simulink model "PMSM_CascadedMPC"  (R2025b)
settings: Solver=ode3  StartTime=0.0  StopTime=12  FixedStep=5e-6  MaxStep=1e-4  RelTol=1e-3
PreLoadFcn:
  | run('params_pmsm_inverter')
undefined symbols (not defined in the file): B_fric, J, Ld, Lq, pp, PsiPM, Rs, Ts_ctrl, Ts_sim, Vdc
libraries: nesl_utility x16, fl_lib x11, ee_lib x8, simulink x1, sdl_lib x1
(part 2 of 2)

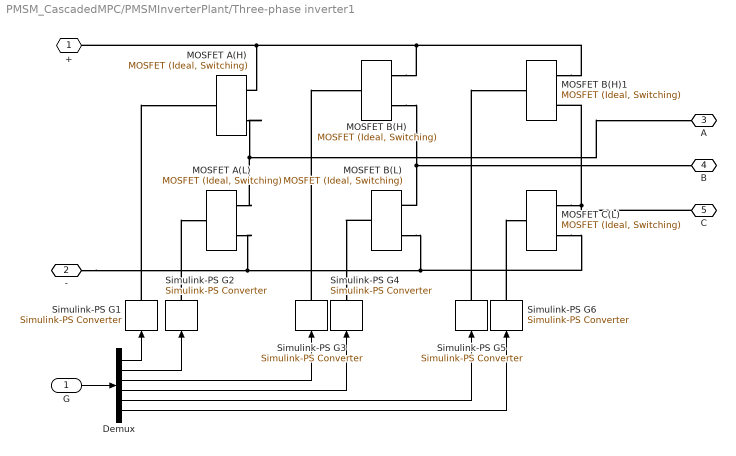
== system PMSM_CascadedMPC/PMSMInverterPlant/Three-phase inverter1 ==
  G : Inport
  Demux : Demux  Outputs=6
  MOSFET A(H) : ee_lib/Semiconductors & Converters/MOSFET (Ideal, Switching)  port_option=ee.enum.controlport.ps  Rds=0.01 Ohm  Goff=1e-6 1/Ohm  Vth=0.5 V  diode_param=ee.enum.semiconductors.protectionDiode.nodynamics  diode_Vf=0.8 V  diode_Ron=0.001 Ohm  diode_Goff=1e-5 1/Ohm  diode_C=50e-9 F  diode_iRM=-235 A  diode_iF=300 A  diode_idot=-50 A/us  diode_trr_param=ee.enum.converters.diodeReverseParam.trr_factor  diode_trr_factor=3  diode_trr=15 us  diode_Qrr=1500 s*uA  ids_specify=off  ids_priority=None  ids=0 A  ids_nominal_specify=off  ids_nominal_value=1  ids_nominal_unit=A  vds_specify=off  vds_priority=None  vds=0 V  vds_nominal_specify=off  vds_nominal_value=1  vds_nominal_unit=V  vgs_specify=off  vgs_priority=None  vgs=0 V  vgs_nominal_specify=off  vgs_nominal_value=1  vgs_nominal_unit=V  thermal_loss_option=ee.enum.converters.thermalLossOption.constantvalues  Von_data=[0, 1.8, 3.2, 6, 10, 16; 0, 2, 5.5, 9.5, 15, 25] V  Tj=[298.15, 448.15] K  Iout_data=[0, 20, 40, 60, 80, 100] A  Eon_data=[0, 55.04, 124.57, 235.53, 362.12; 0, 71.25, 161.25, 304.88, 468.75] * 1e-6 J  Eoff_data=[0, 18, 30, 56.1, 76.5; 0, 22.5, 37.5, 70.13, 95.63] * 1e-6 J  Eon_data_3D=[zeros(2, 5, 3)] J  Eoff_data_3D=[zeros(2, 5, 3)] J  Tj_loss=[298.15, 448.15] K  Iout_data_loss=[0, 10, 20, 30, 40] A  tabulateWithVds=false  Vds_loss=[0, 150, 300] V  Eon_scalar=22.86e-3 J  Eoff_scalar=17.14e-3 J  Voff=800 V  Iout_scalar=600 A  useCurrentFromPreviousCycle=false  useVoltageFromPreviousCycle=false  diodeModelType=ee.enum.converters.diodeModelType.pwl  diodeTableType=ee.enum.diode.tableType.IfMat  diode_ReverseIVType=ee.enum.diode.diodeReverseIV.constant  diode_IfMat=[.07, .12, .19, 1.75, 4.24, 7.32, 11.2; .16, .3, .72, 2.14, 4.02, 6.35, 9.12] A  diode_VfMat=[.9, 1.15, 1.25, 1.5, 1.75, 2.17, 2.6, 2.85; .58, .68, .75, 1.1, 1.38, 1.77, 2.27, 2.7] V  diode_TjVec=[25, 125] degC  diode_VfVec=[.5, .7, .9, 1.3, 1.7, 2.1, 2.5] V  diode_IfVec=[.1, .2, .5, 1, 2, 4, 7, 10] A  diode_IrMat=[1e-06, 2e-06, 5e-06, 1e-05, 2.5e-05, 5e-05, .0001; 2e-06, 5e-06, 1e-05, 4e-05, 8e-05, .0002, .0005] A  diode_VrMat=[10, 100, 200, 250, 300, 325, 350; 10, 70, 160, 220, 270, 300, 320] V  diode_VrVec=[10, 20, 40, 50, 70, 80, 100] V  diode_IrVec=[1e-06, 2e-06, 5e-06, 1e-05, 2e-05, 5e-05, .0001] A  diode_Vr=-600 V  diode_Ls=150 nH  diode_Erec=0.03 J  diode_rec_loss_model=ee.enum.diode.reverseRecoveryModel.fixed  diode_ErecVal=0 J  diode_scaleWithIandV=true  diode_ErecMat=zeros(2, 3) J  diode_TjrecVec=[298.15, 398.15] K  diode_IfrecVec=[.1, 1, 10] A  diode_IrecVal=10 A  diode_VrecVal=10 V  diode_tFilter=1 / 1000 / 100 s  separateThermalPortForDiode=false  thermal_network_parameterization=ee.enum.thermalNetworkTopology.junctionCase  Rth=[.03, .2] K/W  Rth_Cauer=[.03, .1, .2] K/W  Rth_Foster=[.08, .14, .22, .16] K/W  thermal_mass_parameterization=ee.enum.thermalNetwork.thermalmass  thermal_mass=[3, 25] J/K  thermal_mass_Cauer=[3, 10, 25] J/K  thermal_mass_Foster=[.001, .005, .05, .5] J/K  thermal_time_constant=[.1, 5] s  thermal_time_constant_Cauer=[.1, 1, 5] s  thermal_time_constant_Foster=[7e-05, .0007, .01, .08] s  thermal_mass_initial_temperatures=[25, 25] degC  thermal_mass_initial_temperatures_Cauer=[25, 25, 25] degC  junction_thermal_mass=5 J/K  Tvec_initial_Foster=[25, 25, 25, 25] degC  RthDiode=[.03, .2] K/W  RthCauerDiode=[.03, .1, .2] K/W  RthFosterDiode=[.03, .2] K/W  thermalMassDiode=[3, 25] J/K  thermalMassCauerDiode=[3, 10, 25] J/K  thermalMassFosterDiode=[33, 50] J/K  thermalTauDiode=[.1, 5] s  thermalTauCauerDiode=[.1, 1, 5] s  thermalTauFosterDiode=[1, 10] s  thermalMassInitTempDiode=[25, 25] degC  thermalMassInitTempCauerDiode=[25, 25, 25] degC  junctionthermalMassDiode=0.1 J/K  TVecInitialFosterDiode=[25, 25, 25, 25] degC  no_thermal_network=0  mosfet_junction_temperature_specify=on  mosfet_junction_temperature_priority=None  mosfet_junction_temperature=25 degC  mosfet_junction_temperature_nominal_specify=off  mosfet_junction_temperature_nominal_value=1  mosfet_junction_temperature_nominal_unit=degC  diode_junction_temperature_specify=off  diode_junction_temperature_priority=None  diode_junction_temperature=25 degC  diode_junction_temperature_nominal_specify=off  diode_junction_temperature_nominal_value=1  diode_junction_temperature_nominal_unit=degC  Qj_specify=off  Qj_priority=None  Qj=0 W  Qj_nominal_specify=off  Qj_nominal_value=1  Qj_nominal_unit=W  accumulatedSwitchingLosses_specify=off  accumulatedSwitchingLosses_priority=None  accumulatedSwitchingLosses=0 J
  MOSFET A(L) : ee_lib/Semiconductors & Converters/MOSFET (Ideal, Switching)  port_option=ee.enum.controlport.ps  Rds=0.01 Ohm  Goff=1e-6 1/Ohm  Vth=0.5 V  diode_param=ee.enum.semiconductors.protectionDiode.nodynamics  diode_Vf=0.8 V  diode_Ron=0.001 Ohm  diode_Goff=1e-5 1/Ohm  diode_C=50e-9 F  diode_iRM=-235 A  diode_iF=300 A  diode_idot=-50 A/us  diode_trr_param=ee.enum.converters.diodeReverseParam.trr_factor  diode_trr_factor=3  diode_trr=15 us  diode_Qrr=1500 s*uA  ids_specify=off  ids_priority=None  ids=0 A  ids_nominal_specify=off  ids_nominal_value=1  ids_nominal_unit=A  vds_specify=off  vds_priority=None  vds=0 V  vds_nominal_specify=off  vds_nominal_value=1  vds_nominal_unit=V  vgs_specify=off  vgs_priority=None  vgs=0 V  vgs_nominal_specify=off  vgs_nominal_value=1  vgs_nominal_unit=V  thermal_loss_option=ee.enum.converters.thermalLossOption.constantvalues  Von_data=[0, 1.8, 3.2, 6, 10, 16; 0, 2, 5.5, 9.5, 15, 25] V  Tj=[298.15, 448.15] K  Iout_data=[0, 20, 40, 60, 80, 100] A  Eon_data=[0, 55.04, 124.57, 235.53, 362.12; 0, 71.25, 161.25, 304.88, 468.75] * 1e-6 J  Eoff_data=[0, 18, 30, 56.1, 76.5; 0, 22.5, 37.5, 70.13, 95.63] * 1e-6 J  Eon_data_3D=[zeros(2, 5, 3)] J  Eoff_data_3D=[zeros(2, 5, 3)] J  Tj_loss=[298.15, 448.15] K  Iout_data_loss=[0, 10, 20, 30, 40] A  tabulateWithVds=false  Vds_loss=[0, 150, 300] V  Eon_scalar=22.86e-3 J  Eoff_scalar=17.14e-3 J  Voff=300 V  Iout_scalar=600 A  useCurrentFromPreviousCycle=false  useVoltageFromPreviousCycle=false  diodeModelType=ee.enum.converters.diodeModelType.pwl  diodeTableType=ee.enum.diode.tableType.IfMat  diode_ReverseIVType=ee.enum.diode.diodeReverseIV.constant  diode_IfMat=[.07, .12, .19, 1.75, 4.24, 7.32, 11.2; .16, .3, .72, 2.14, 4.02, 6.35, 9.12] A  diode_VfMat=[.9, 1.15, 1.25, 1.5, 1.75, 2.17, 2.6, 2.85; .58, .68, .75, 1.1, 1.38, 1.77, 2.27, 2.7] V  diode_TjVec=[25, 125] degC  diode_VfVec=[.5, .7, .9, 1.3, 1.7, 2.1, 2.5] V  diode_IfVec=[.1, .2, .5, 1, 2, 4, 7, 10] A  diode_IrMat=[1e-06, 2e-06, 5e-06, 1e-05, 2.5e-05, 5e-05, .0001; 2e-06, 5e-06, 1e-05, 4e-05, 8e-05, .0002, .0005] A  diode_VrMat=[10, 100, 200, 250, 300, 325, 350; 10, 70, 160, 220, 270, 300, 320] V  diode_VrVec=[10, 20, 40, 50, 70, 80, 100] V  diode_IrVec=[1e-06, 2e-06, 5e-06, 1e-05, 2e-05, 5e-05, .0001] A  diode_Vr=-600 V  diode_Ls=150 nH  diode_Erec=0.03 J  diode_rec_loss_model=ee.enum.diode.reverseRecoveryModel.fixed  diode_ErecVal=0 J  diode_scaleWithIandV=true  diode_ErecMat=zeros(2, 3) J  diode_TjrecVec=[298.15, 398.15] K  diode_IfrecVec=[.1, 1, 10] A  diode_IrecVal=10 A  diode_VrecVal=10 V  diode_tFilter=1 / 1000 / 100 s  separateThermalPortForDiode=false  thermal_network_parameterization=ee.enum.thermalNetworkTopology.external  Rth=[.03, .2] K/W  Rth_Cauer=[.03, .1, .2] K/W  Rth_Foster=[.08, .14, .22, .16] K/W  thermal_mass_parameterization=ee.enum.thermalNetwork.timeconstant  thermal_mass=[3, 25] J/K  thermal_mass_Cauer=[3, 10, 25] J/K  thermal_mass_Foster=[.001, .005, .05, .5] J/K  thermal_time_constant=[.1, 5] s  thermal_time_constant_Cauer=[.1, 1, 5] s  thermal_time_constant_Foster=[7e-05, .0007, .01, .08] s  thermal_mass_initial_temperatures=[25, 25] degC  thermal_mass_initial_temperatures_Cauer=[25, 25, 25] degC  junction_thermal_mass=0.1 J/K  Tvec_initial_Foster=[25, 25, 25, 25] degC  RthDiode=[.03, .2] K/W  RthCauerDiode=[.03, .1, .2] K/W  RthFosterDiode=[.03, .2] K/W  thermalMassDiode=[3, 25] J/K  thermalMassCauerDiode=[3, 10, 25] J/K  thermalMassFosterDiode=[33, 50] J/K  thermalTauDiode=[.1, 5] s  thermalTauCauerDiode=[.1, 1, 5] s  thermalTauFosterDiode=[1, 10] s  thermalMassInitTempDiode=[25, 25] degC  thermalMassInitTempCauerDiode=[25, 25, 25] degC  junctionthermalMassDiode=0.1 J/K  TVecInitialFosterDiode=[25, 25, 25, 25] degC  no_thermal_network=0  mosfet_junction_temperature_specify=off  mosfet_junction_temperature_priority=None  mosfet_junction_temperature=25 degC  mosfet_junction_temperature_nominal_specify=off  mosfet_junction_temperature_nominal_value=1  mosfet_junction_temperature_nominal_unit=degC  diode_junction_temperature_specify=off  diode_junction_temperature_priority=None  diode_junction_temperature=25 degC  diode_junction_temperature_nominal_specify=off  diode_junction_temperature_nominal_value=1  diode_junction_temperature_nominal_unit=degC  Qj_specify=off  Qj_priority=None  Qj=0 W  Qj_nominal_specify=off  Qj_nominal_value=1  Qj_nominal_unit=W  accumulatedSwitchingLosses_specify=off  accumulatedSwitchingLosses_priority=None  accumulatedSwitchingLosses=0 J
  MOSFET B(H) : ee_lib/Semiconductors & Converters/MOSFET (Ideal, Switching)  port_option=ee.enum.controlport.ps  Rds=0.01 Ohm  Goff=1e-6 1/Ohm  Vth=0.5 V  diode_param=ee.enum.semiconductors.protectionDiode.nodynamics  diode_Vf=0.8 V  diode_Ron=0.001 Ohm  diode_Goff=1e-5 1/Ohm  diode_C=50e-9 F  diode_iRM=-235 A  diode_iF=300 A  diode_idot=-50 A/us  diode_trr_param=ee.enum.converters.diodeReverseParam.trr_factor  diode_trr_factor=3  diode_trr=15 us  diode_Qrr=1500 s*uA  ids_specify=off  ids_priority=None  ids=0 A  ids_nominal_specify=off  ids_nominal_value=1  ids_nominal_unit=A  vds_specify=off  vds_priority=None  vds=0 V  vds_nominal_specify=off  vds_nominal_value=1  vds_nominal_unit=V  vgs_specify=off  vgs_priority=None  vgs=0 V  vgs_nominal_specify=off  vgs_nominal_value=1  vgs_nominal_unit=V  thermal_loss_option=ee.enum.converters.thermalLossOption.constantvalues  Von_data=[0, 1.8, 3.2, 6, 10, 16; 0, 2, 5.5, 9.5, 15, 25] V  Tj=[298.15, 448.15] K  Iout_data=[0, 20, 40, 60, 80, 100] A  Eon_data=[0, 55.04, 124.57, 235.53, 362.12; 0, 71.25, 161.25, 304.88, 468.75] * 1e-6 J  Eoff_data=[0, 18, 30, 56.1, 76.5; 0, 22.5, 37.5, 70.13, 95.63] * 1e-6 J  Eon_data_3D=[zeros(2, 5, 3)] J  Eoff_data_3D=[zeros(2, 5, 3)] J  Tj_loss=[298.15, 448.15] K  Iout_data_loss=[0, 10, 20, 30, 40] A  tabulateWithVds=false  Vds_loss=[0, 150, 300] V  Eon_scalar=22.86e-3 J  Eoff_scalar=17.14e-3 J  Voff=300 V  Iout_scalar=600 A  useCurrentFromPreviousCycle=false  useVoltageFromPreviousCycle=false  diodeModelType=ee.enum.converters.diodeModelType.pwl  diodeTableType=ee.enum.diode.tableType.IfMat  diode_ReverseIVType=ee.enum.diode.diodeReverseIV.constant  diode_IfMat=[.07, .12, .19, 1.75, 4.24, 7.32, 11.2; .16, .3, .72, 2.14, 4.02, 6.35, 9.12] A  diode_VfMat=[.9, 1.15, 1.25, 1.5, 1.75, 2.17, 2.6, 2.85; .58, .68, .75, 1.1, 1.38, 1.77, 2.27, 2.7] V  diode_TjVec=[25, 125] degC  diode_VfVec=[.5, .7, .9, 1.3, 1.7, 2.1, 2.5] V  diode_IfVec=[.1, .2, .5, 1, 2, 4, 7, 10] A  diode_IrMat=[1e-06, 2e-06, 5e-06, 1e-05, 2.5e-05, 5e-05, .0001; 2e-06, 5e-06, 1e-05, 4e-05, 8e-05, .0002, .0005] A  diode_VrMat=[10, 100, 200, 250, 300, 325, 350; 10, 70, 160, 220, 270, 300, 320] V  diode_VrVec=[10, 20, 40, 50, 70, 80, 100] V  diode_IrVec=[1e-06, 2e-06, 5e-06, 1e-05, 2e-05, 5e-05, .0001] A  diode_Vr=-600 V  diode_Ls=150 nH  diode_Erec=0.03 J  diode_rec_loss_model=ee.enum.diode.reverseRecoveryModel.fixed  diode_ErecVal=0 J  diode_scaleWithIandV=true  diode_ErecMat=zeros(2, 3) J  diode_TjrecVec=[298.15, 398.15] K  diode_IfrecVec=[.1, 1, 10] A  diode_IrecVal=10 A  diode_VrecVal=10 V  diode_tFilter=1 / 1000 / 100 s  separateThermalPortForDiode=false  thermal_network_parameterization=ee.enum.thermalNetworkTopology.external  Rth=[.03, .2] K/W  Rth_Cauer=[.03, .1, .2] K/W  Rth_Foster=[.08, .14, .22, .16] K/W  thermal_mass_parameterization=ee.enum.thermalNetwork.timeconstant  thermal_mass=[3, 25] J/K  thermal_mass_Cauer=[3, 10, 25] J/K  thermal_mass_Foster=[.001, .005, .05, .5] J/K  thermal_time_constant=[.1, 5] s  thermal_time_constant_Cauer=[.1, 1, 5] s  thermal_time_constant_Foster=[7e-05, .0007, .01, .08] s  thermal_mass_initial_temperatures=[25, 25] degC  thermal_mass_initial_temperatures_Cauer=[25, 25, 25] degC  junction_thermal_mass=0.1 J/K  Tvec_initial_Foster=[25, 25, 25, 25] degC  RthDiode=[.03, .2] K/W  RthCauerDiode=[.03, .1, .2] K/W  RthFosterDiode=[.03, .2] K/W  thermalMassDiode=[3, 25] J/K  thermalMassCauerDiode=[3, 10, 25] J/K  thermalMassFosterDiode=[33, 50] J/K  thermalTauDiode=[.1, 5] s  thermalTauCauerDiode=[.1, 1, 5] s  thermalTauFosterDiode=[1, 10] s  thermalMassInitTempDiode=[25, 25] degC  thermalMassInitTempCauerDiode=[25, 25, 25] degC  junctionthermalMassDiode=0.1 J/K  TVecInitialFosterDiode=[25, 25, 25, 25] degC  no_thermal_network=0  mosfet_junction_temperature_specify=off  mosfet_junction_temperature_priority=None  mosfet_junction_temperature=25 degC  mosfet_junction_temperature_nominal_specify=off  mosfet_junction_temperature_nominal_value=1  mosfet_junction_temperature_nominal_unit=degC  diode_junction_temperature_specify=off  diode_junction_temperature_priority=None  diode_junction_temperature=25 degC  diode_junction_temperature_nominal_specify=off  diode_junction_temperature_nominal_value=1  diode_junction_temperature_nominal_unit=degC  Qj_specify=off  Qj_priority=None  Qj=0 W  Qj_nominal_specify=off  Qj_nominal_value=1  Qj_nominal_unit=W  accumulatedSwitchingLosses_specify=off  accumulatedSwitchingLosses_priority=None  accumulatedSwitchingLosses=0 J
  MOSFET B(H)1 : ee_lib/Semiconductors & Converters/MOSFET (Ideal, Switching)  port_option=ee.enum.controlport.ps  Rds=0.01 Ohm  Goff=1e-6 1/Ohm  Vth=0.5 V  diode_param=ee.enum.semiconductors.protectionDiode.nodynamics  diode_Vf=0.8 V  diode_Ron=0.001 Ohm  diode_Goff=1e-5 1/Ohm  diode_C=50e-9 F  diode_iRM=-235 A  diode_iF=300 A  diode_idot=-50 A/us  diode_trr_param=ee.enum.converters.diodeReverseParam.trr_factor  diode_trr_factor=3  diode_trr=15 us  diode_Qrr=1500 s*uA  ids_specify=off  ids_priority=None  ids=0 A  ids_nominal_specify=off  ids_nominal_value=1  ids_nominal_unit=A  vds_specify=off  vds_priority=None  vds=0 V  vds_nominal_specify=off  vds_nominal_value=1  vds_nominal_unit=V  vgs_specify=off  vgs_priority=None  vgs=0 V  vgs_nominal_specify=off  vgs_nominal_value=1  vgs_nominal_unit=V  thermal_loss_option=ee.enum.converters.thermalLossOption.constantvalues  Von_data=[0, 1.8, 3.2, 6, 10, 16; 0, 2, 5.5, 9.5, 15, 25] V  Tj=[298.15, 448.15] K  Iout_data=[0, 20, 40, 60, 80, 100] A  Eon_data=[0, 55.04, 124.57, 235.53, 362.12; 0, 71.25, 161.25, 304.88, 468.75] * 1e-6 J  Eoff_data=[0, 18, 30, 56.1, 76.5; 0, 22.5, 37.5, 70.13, 95.63] * 1e-6 J  Eon_data_3D=[zeros(2, 5, 3)] J  Eoff_data_3D=[zeros(2, 5, 3)] J  Tj_loss=[298.15, 448.15] K  Iout_data_loss=[0, 10, 20, 30, 40] A  tabulateWithVds=false  Vds_loss=[0, 150, 300] V  Eon_scalar=22.86e-3 J  Eoff_scalar=17.14e-3 J  Voff=300 V  Iout_scalar=600 A  useCurrentFromPreviousCycle=false  useVoltageFromPreviousCycle=false  diodeModelType=ee.enum.converters.diodeModelType.pwl  diodeTableType=ee.enum.diode.tableType.IfMat  diode_ReverseIVType=ee.enum.diode.diodeReverseIV.constant  diode_IfMat=[.07, .12, .19, 1.75, 4.24, 7.32, 11.2; .16, .3, .72, 2.14, 4.02, 6.35, 9.12] A  diode_VfMat=[.9, 1.15, 1.25, 1.5, 1.75, 2.17, 2.6, 2.85; .58, .68, .75, 1.1, 1.38, 1.77, 2.27, 2.7] V  diode_TjVec=[25, 125] degC  diode_VfVec=[.5, .7, .9, 1.3, 1.7, 2.1, 2.5] V  diode_IfVec=[.1, .2, .5, 1, 2, 4, 7, 10] A  diode_IrMat=[1e-06, 2e-06, 5e-06, 1e-05, 2.5e-05, 5e-05, .0001; 2e-06, 5e-06, 1e-05, 4e-05, 8e-05, .0002, .0005] A  diode_VrMat=[10, 100, 200, 250, 300, 325, 350; 10, 70, 160, 220, 270, 300, 320] V  diode_VrVec=[10, 20, 40, 50, 70, 80, 100] V  diode_IrVec=[1e-06, 2e-06, 5e-06, 1e-05, 2e-05, 5e-05, .0001] A  diode_Vr=-600 V  diode_Ls=150 nH  diode_Erec=0.03 J  diode_rec_loss_model=ee.enum.diode.reverseRecoveryModel.fixed  diode_ErecVal=0 J  diode_scaleWithIandV=true  diode_ErecMat=zeros(2, 3) J  diode_TjrecVec=[298.15, 398.15] K  diode_IfrecVec=[.1, 1, 10] A  diode_IrecVal=10 A  diode_VrecVal=10 V  diode_tFilter=1 / 1000 / 100 s  separateThermalPortForDiode=false  thermal_network_parameterization=ee.enum.thermalNetworkTopology.external  Rth=[.03, .2] K/W  Rth_Cauer=[.03, .1, .2] K/W  Rth_Foster=[.08, .14, .22, .16] K/W  thermal_mass_parameterization=ee.enum.thermalNetwork.timeconstant  thermal_mass=[3, 25] J/K  thermal_mass_Cauer=[3, 10, 25] J/K  thermal_mass_Foster=[.001, .005, .05, .5] J/K  thermal_time_constant=[.1, 5] s  thermal_time_constant_Cauer=[.1, 1, 5] s  thermal_time_constant_Foster=[7e-05, .0007, .01, .08] s  thermal_mass_initial_temperatures=[25, 25] degC  thermal_mass_initial_temperatures_Cauer=[25, 25, 25] degC  junction_thermal_mass=0.1 J/K  Tvec_initial_Foster=[25, 25, 25, 25] degC  RthDiode=[.03, .2] K/W  RthCauerDiode=[.03, .1, .2] K/W  RthFosterDiode=[.03, .2] K/W  thermalMassDiode=[3, 25] J/K  thermalMassCauerDiode=[3, 10, 25] J/K  thermalMassFosterDiode=[33, 50] J/K  thermalTauDiode=[.1, 5] s  thermalTauCauerDiode=[.1, 1, 5] s  thermalTauFosterDiode=[1, 10] s  thermalMassInitTempDiode=[25, 25] degC  thermalMassInitTempCauerDiode=[25, 25, 25] degC  junctionthermalMassDiode=0.1 J/K  TVecInitialFosterDiode=[25, 25, 25, 25] degC  no_thermal_network=0  mosfet_junction_temperature_specify=off  mosfet_junction_temperature_priority=None  mosfet_junction_temperature=25 degC  mosfet_junction_temperature_nominal_specify=off  mosfet_junction_temperature_nominal_value=1  mosfet_junction_temperature_nominal_unit=degC  diode_junction_temperature_specify=off  diode_junction_temperature_priority=None  diode_junction_temperature=25 degC  diode_junction_temperature_nominal_specify=off  diode_junction_temperature_nominal_value=1  diode_junction_temperature_nominal_unit=degC  Qj_specify=off  Qj_priority=None  Qj=0 W  Qj_nominal_specify=off  Qj_nominal_value=1  Qj_nominal_unit=W  accumulatedSwitchingLosses_specify=off  accumulatedSwitchingLosses_priority=None  accumulatedSwitchingLosses=0 J
  MOSFET B(L) : ee_lib/Semiconductors & Converters/MOSFET (Ideal, Switching)  port_option=ee.enum.controlport.ps  Rds=0.01 Ohm  Goff=1e-6 1/Ohm  Vth=0.5 V  diode_param=ee.enum.semiconductors.protectionDiode.nodynamics  diode_Vf=0.8 V  diode_Ron=0.001 Ohm  diode_Goff=1e-5 1/Ohm  diode_C=50e-9 F  diode_iRM=-235 A  diode_iF=300 A  diode_idot=-50 A/us  diode_trr_param=ee.enum.converters.diodeReverseParam.trr_factor  diode_trr_factor=3  diode_trr=15 us  diode_Qrr=1500 s*uA  ids_specify=off  ids_priority=None  ids=0 A  ids_nominal_specify=off  ids_nominal_value=1  ids_nominal_unit=A  vds_specify=off  vds_priority=None  vds=0 V  vds_nominal_specify=off  vds_nominal_value=1  vds_nominal_unit=V  vgs_specify=off  vgs_priority=None  vgs=0 V  vgs_nominal_specify=off  vgs_nominal_value=1  vgs_nominal_unit=V  thermal_loss_option=ee.enum.converters.thermalLossOption.constantvalues  Von_data=[0, 1.8, 3.2, 6, 10, 16; 0, 2, 5.5, 9.5, 15, 25] V  Tj=[298.15, 448.15] K  Iout_data=[0, 20, 40, 60, 80, 100] A  Eon_data=[0, 55.04, 124.57, 235.53, 362.12; 0, 71.25, 161.25, 304.88, 468.75] * 1e-6 J  Eoff_data=[0, 18, 30, 56.1, 76.5; 0, 22.5, 37.5, 70.13, 95.63] * 1e-6 J  Eon_data_3D=[zeros(2, 5, 3)] J  Eoff_data_3D=[zeros(2, 5, 3)] J  Tj_loss=[298.15, 448.15] K  Iout_data_loss=[0, 10, 20, 30, 40] A  tabulateWithVds=false  Vds_loss=[0, 150, 300] V  Eon_scalar=22.86e-3 J  Eoff_scalar=17.14e-3 J  Voff=300 V  Iout_scalar=600 A  useCurrentFromPreviousCycle=false  useVoltageFromPreviousCycle=false  diodeModelType=ee.enum.converters.diodeModelType.pwl  diodeTableType=ee.enum.diode.tableType.IfMat  diode_ReverseIVType=ee.enum.diode.diodeReverseIV.constant  diode_IfMat=[.07, .12, .19, 1.75, 4.24, 7.32, 11.2; .16, .3, .72, 2.14, 4.02, 6.35, 9.12] A  diode_VfMat=[.9, 1.15, 1.25, 1.5, 1.75, 2.17, 2.6, 2.85; .58, .68, .75, 1.1, 1.38, 1.77, 2.27, 2.7] V  diode_TjVec=[25, 125] degC  diode_VfVec=[.5, .7, .9, 1.3, 1.7, 2.1, 2.5] V  diode_IfVec=[.1, .2, .5, 1, 2, 4, 7, 10] A  diode_IrMat=[1e-06, 2e-06, 5e-06, 1e-05, 2.5e-05, 5e-05, .0001; 2e-06, 5e-06, 1e-05, 4e-05, 8e-05, .0002, .0005] A  diode_VrMat=[10, 100, 200, 250, 300, 325, 350; 10, 70, 160, 220, 270, 300, 320] V  diode_VrVec=[10, 20, 40, 50, 70, 80, 100] V  diode_IrVec=[1e-06, 2e-06, 5e-06, 1e-05, 2e-05, 5e-05, .0001] A  diode_Vr=-600 V  diode_Ls=150 nH  diode_Erec=0.03 J  diode_rec_loss_model=ee.enum.diode.reverseRecoveryModel.fixed  diode_ErecVal=0 J  diode_scaleWithIandV=true  diode_ErecMat=zeros(2, 3) J  diode_TjrecVec=[298.15, 398.15] K  diode_IfrecVec=[.1, 1, 10] A  diode_IrecVal=10 A  diode_VrecVal=10 V  diode_tFilter=1 / 1000 / 100 s  separateThermalPortForDiode=false  thermal_network_parameterization=ee.enum.thermalNetworkTopology.external  Rth=[.03, .2] K/W  Rth_Cauer=[.03, .1, .2] K/W  Rth_Foster=[.08, .14, .22, .16] K/W  thermal_mass_parameterization=ee.enum.thermalNetwork.timeconstant  thermal_mass=[3, 25] J/K  thermal_mass_Cauer=[3, 10, 25] J/K  thermal_mass_Foster=[.001, .005, .05, .5] J/K  thermal_time_constant=[.1, 5] s  thermal_time_constant_Cauer=[.1, 1, 5] s  thermal_time_constant_Foster=[7e-05, .0007, .01, .08] s  thermal_mass_initial_temperatures=[25, 25] degC  thermal_mass_initial_temperatures_Cauer=[25, 25, 25] degC  junction_thermal_mass=0.1 J/K  Tvec_initial_Foster=[25, 25, 25, 25] degC  RthDiode=[.03, .2] K/W  RthCauerDiode=[.03, .1, .2] K/W  RthFosterDiode=[.03, .2] K/W  thermalMassDiode=[3, 25] J/K  thermalMassCauerDiode=[3, 10, 25] J/K  thermalMassFosterDiode=[33, 50] J/K  thermalTauDiode=[.1, 5] s  thermalTauCauerDiode=[.1, 1, 5] s  thermalTauFosterDiode=[1, 10] s  thermalMassInitTempDiode=[25, 25] degC  thermalMassInitTempCauerDiode=[25, 25, 25] degC  junctionthermalMassDiode=0.1 J/K  TVecInitialFosterDiode=[25, 25, 25, 25] degC  no_thermal_network=0  mosfet_junction_temperature_specify=off  mosfet_junction_temperature_priority=None  mosfet_junction_temperature=25 degC  mosfet_junction_temperature_nominal_specify=off  mosfet_junction_temperature_nominal_value=1  mosfet_junction_temperature_nominal_unit=degC  diode_junction_temperature_specify=off  diode_junction_temperature_priority=None  diode_junction_temperature=25 degC  diode_junction_temperature_nominal_specify=off  diode_junction_temperature_nominal_value=1  diode_junction_temperature_nominal_unit=degC  Qj_specify=off  Qj_priority=None  Qj=0 W  Qj_nominal_specify=off  Qj_nominal_value=1  Qj_nominal_unit=W  accumulatedSwitchingLosses_specify=off  accumulatedSwitchingLosses_priority=None  accumulatedSwitchingLosses=0 J
  MOSFET C(L) : ee_lib/Semiconductors & Converters/MOSFET (Ideal, Switching)  port_option=ee.enum.controlport.ps  Rds=0.01 Ohm  Goff=1e-6 1/Ohm  Vth=0.5 V  diode_param=ee.enum.semiconductors.protectionDiode.nodynamics  diode_Vf=0.8 V  diode_Ron=0.001 Ohm  diode_Goff=1e-5 1/Ohm  diode_C=50e-9 F  diode_iRM=-235 A  diode_iF=300 A  diode_idot=-50 A/us  diode_trr_param=ee.enum.converters.diodeReverseParam.trr_factor  diode_trr_factor=3  diode_trr=15 us  diode_Qrr=1500 s*uA  ids_specify=off  ids_priority=None  ids=0 A  ids_nominal_specify=off  ids_nominal_value=1  ids_nominal_unit=A  vds_specify=off  vds_priority=None  vds=0 V  vds_nominal_specify=off  vds_nominal_value=1  vds_nominal_unit=V  vgs_specify=off  vgs_priority=None  vgs=0 V  vgs_nominal_specify=off  vgs_nominal_value=1  vgs_nominal_unit=V  thermal_loss_option=ee.enum.converters.thermalLossOption.constantvalues  Von_data=[0, 1.8, 3.2, 6, 10, 16; 0, 2, 5.5, 9.5, 15, 25] V  Tj=[298.15, 448.15] K  Iout_data=[0, 20, 40, 60, 80, 100] A  Eon_data=[0, 55.04, 124.57, 235.53, 362.12; 0, 71.25, 161.25, 304.88, 468.75] * 1e-6 J  Eoff_data=[0, 18, 30, 56.1, 76.5; 0, 22.5, 37.5, 70.13, 95.63] * 1e-6 J  Eon_data_3D=[zeros(2, 5, 3)] J  Eoff_data_3D=[zeros(2, 5, 3)] J  Tj_loss=[298.15, 448.15] K  Iout_data_loss=[0, 10, 20, 30, 40] A  tabulateWithVds=false  Vds_loss=[0, 150, 300] V  Eon_scalar=22.86e-3 J  Eoff_scalar=17.14e-3 J  Voff=300 V  Iout_scalar=600 A  useCurrentFromPreviousCycle=false  useVoltageFromPreviousCycle=false  diodeModelType=ee.enum.converters.diodeModelType.pwl  diodeTableType=ee.enum.diode.tableType.IfMat  diode_ReverseIVType=ee.enum.diode.diodeReverseIV.constant  diode_IfMat=[.07, .12, .19, 1.75, 4.24, 7.32, 11.2; .16, .3, .72, 2.14, 4.02, 6.35, 9.12] A  diode_VfMat=[.9, 1.15, 1.25, 1.5, 1.75, 2.17, 2.6, 2.85; .58, .68, .75, 1.1, 1.38, 1.77, 2.27, 2.7] V  diode_TjVec=[25, 125] degC  diode_VfVec=[.5, .7, .9, 1.3, 1.7, 2.1, 2.5] V  diode_IfVec=[.1, .2, .5, 1, 2, 4, 7, 10] A  diode_IrMat=[1e-06, 2e-06, 5e-06, 1e-05, 2.5e-05, 5e-05, .0001; 2e-06, 5e-06, 1e-05, 4e-05, 8e-05, .0002, .0005] A  diode_VrMat=[10, 100, 200, 250, 300, 325, 350; 10, 70, 160, 220, 270, 300, 320] V  diode_VrVec=[10, 20, 40, 50, 70, 80, 100] V  diode_IrVec=[1e-06, 2e-06, 5e-06, 1e-05, 2e-05, 5e-05, .0001] A  diode_Vr=-600 V  diode_Ls=150 nH  diode_Erec=0.03 J  diode_rec_loss_model=ee.enum.diode.reverseRecoveryModel.fixed  diode_ErecVal=0 J  diode_scaleWithIandV=true  diode_ErecMat=zeros(2, 3) J  diode_TjrecVec=[298.15, 398.15] K  diode_IfrecVec=[.1, 1, 10] A  diode_IrecVal=10 A  diode_VrecVal=10 V  diode_tFilter=1 / 1000 / 100 s  separateThermalPortForDiode=false  thermal_network_parameterization=ee.enum.thermalNetworkTopology.external  Rth=[.03, .2] K/W  Rth_Cauer=[.03, .1, .2] K/W  Rth_Foster=[.08, .14, .22, .16] K/W  thermal_mass_parameterization=ee.enum.thermalNetwork.timeconstant  thermal_mass=[3, 25] J/K  thermal_mass_Cauer=[3, 10, 25] J/K  thermal_mass_Foster=[.001, .005, .05, .5] J/K  thermal_time_constant=[.1, 5] s  thermal_time_constant_Cauer=[.1, 1, 5] s  thermal_time_constant_Foster=[7e-05, .0007, .01, .08] s  thermal_mass_initial_temperatures=[25, 25] degC  thermal_mass_initial_temperatures_Cauer=[25, 25, 25] degC  junction_thermal_mass=0.1 J/K  Tvec_initial_Foster=[25, 25, 25, 25] degC  RthDiode=[.03, .2] K/W  RthCauerDiode=[.03, .1, .2] K/W  RthFosterDiode=[.03, .2] K/W  thermalMassDiode=[3, 25] J/K  thermalMassCauerDiode=[3, 10, 25] J/K  thermalMassFosterDiode=[33, 50] J/K  thermalTauDiode=[.1, 5] s  thermalTauCauerDiode=[.1, 1, 5] s  thermalTauFosterDiode=[1, 10] s  thermalMassInitTempDiode=[25, 25] degC  thermalMassInitTempCauerDiode=[25, 25, 25] degC  junctionthermalMassDiode=0.1 J/K  TVecInitialFosterDiode=[25, 25, 25, 25] degC  no_thermal_network=0  mosfet_junction_temperature_specify=off  mosfet_junction_temperature_priority=None  mosfet_junction_temperature=25 degC  mosfet_junction_temperature_nominal_specify=off  mosfet_junction_temperature_nominal_value=1  mosfet_junction_temperature_nominal_unit=degC  diode_junction_temperature_specify=off  diode_junction_temperature_priority=None  diode_junction_temperature=25 degC  diode_junction_temperature_nominal_specify=off  diode_junction_temperature_nominal_value=1  diode_junction_temperature_nominal_unit=degC  Qj_specify=off  Qj_priority=None  Qj=0 W  Qj_nominal_specify=off  Qj_nominal_value=1  Qj_nominal_unit=W  accumulatedSwitchingLosses_specify=off  accumulatedSwitchingLosses_priority=None  accumulatedSwitchingLosses=0 J
  Simulink-PS G{1..6} (6 alike) : nesl_utility/Simulink-PS Converter  PhysicalDomain=network_engine_domain  SubClassName=ps_input  LeftPortType=input  RightPortType=output  PseudoPeriodic=off  Frequencies=[]  NoiseDistribution=none  NoiseParameters=[]  Unit=1  AffineConversion=off  FilteringAndDerivatives=zero  SimscapeFilterOrder=1  InputFilterTimeConstant=1e-6  UdotUserProvided=0
  + : PMIOPort  Tag=PMCPort  Side=Left
  - : PMIOPort  Tag=PMCPort  Port=2  Side=Left
  A : PMIOPort  Tag=PMCPort  Port=3  Side=Right
  B : PMIOPort  Tag=PMCPort  Port=4  Side=Right
  C : PMIOPort  Tag=PMCPort  Port=5  Side=Right
  wires:
  Demux/6 -> Simulink-PS G6/1
  Demux/5 -> Simulink-PS G5/1
  Demux/4 -> Simulink-PS G4/1
  Demux/3 -> Simulink-PS G3/1
  Demux/2 -> Simulink-PS G2/1
  G/1 -> Demux/1
  Demux/1 -> Simulink-PS G1/1
  connections:
  MOSFET B(L)/LConn1 -- Simulink-PS G4/RConn1
  -/RConn1 -- MOSFET C(L)/RConn2 -- MOSFET B(L)/RConn2 -- MOSFET A(L)/RConn2
  MOSFET A(H)/RConn2 -- MOSFET A(L)/RConn1 -- A/RConn1
  MOSFET B(H)/RConn2 -- B/RConn1 -- MOSFET B(L)/RConn1
  MOSFET C(L)/RConn1 -- MOSFET B(H)1/RConn2 -- C/RConn1
  MOSFET B(H)1/RConn1 -- MOSFET B(H)/RConn1 -- MOSFET A(H)/RConn1 -- +/RConn1
  Simulink-PS G1/RConn1 -- MOSFET A(H)/LConn1
  Simulink-PS G2/RConn1 -- MOSFET A(L)/LConn1
  Simulink-PS G3/RConn1 -- MOSFET B(H)/LConn1
  Simulink-PS G6/RConn1 -- MOSFET C(L)/LConn1
  Simulink-PS G5/RConn1 -- MOSFET B(H)1/LConn1

== matlab function PMSM_CascadedMPC/CCSMPC_Controller/Speed_MPC ==
  data: w_ref input double size=1; id_ref output double size=1; omega_m input double size=1; Vdc input double size=1; Rs input double size=1; Ld input double size=1; Lq input double size=1; PsiPM input double size=1; iq_ref output double size=1; control_mode input; J_est input; B_est input
function [id_ref, iq_ref] = Outer_MPC(w_ref, omega_m, Vdc, Rs, Ld, Lq, PsiPM, control_mode, J_est, B_est)
    % Cascaded Multi-Rate Speed MPC & Analytical Smooth MTPA/FW Optimizer
    % control_mode: 1 = Active Speed Control, 0/2 = Disabled / Tuning Mode
    
    id_ref = zeros(1, 1, 'double');
    iq_ref = zeros(1, 1, 'double');
    
    pp = 6.0;         % i3 motor pole pairs
    I_max = 565.0;    % Maximum phase current (A peak)
    Ts_dt = 1e-4;     % Discrete sample interval (100 us / 10 kHz)
    
    persistent omega_filt;
    persistent e_int;
    
    if isempty(omega_filt)
        omega_filt = double(omega_m);
        e_int = 0.0;
    end
    
    % Control Mode Bypass during AutoTuning (mode ~= 1)
    if control_mode ~= 1
        omega_filt = double(omega_m);
        e_int = 0.0;
        id_ref(1) = 0.0;
        iq_ref(1) = 0.0;
        return;
    end
    
    % Parameter extraction and protective lower bounds
    J_val = max(double(J_est), 0.001);
    B_val = max(double(B_est), 0.0);
    Psi_val = max(double(PsiPM), 0.005);
    Ld_val = max(double(Ld), 1e-6);
    Lq_val = max(double(Lq), 1e-6);
    dL = Lq_val - Ld_val;
    
    % 1. Low-pass filter raw measured speed to eliminate PWM carrier derivative chatter
    alpha_w = 0.95;
    omega_filt = alpha_w * omega_filt + (1.0 - alpha_w) * double(omega_m);
    
    % Convert to mechanical speed
    w_ref_mech = double(w_ref) / pp;
    w_mech = omega_filt / pp;
    
    % 2. Speed MPC control law (Matched to inertia J)
    e_w = w_ref_mech - w_mech;
    e_int = e_int + e_w * Ts_dt;
    
    Kp_w = 6.5 * (J_val / 0.0867);
    Ki_w = 120.0 * (J_val / 0.0867);
    
    Te_cmd = Kp_w * e_w + Ki_w * e_int + B_val * w_mech;
    
    % Anti-windup clamping
    if Te_cmd > 258.2
        Te_cmd = 258.2;
        e_int = e_int - e_w * Ts_dt;
    elseif Te_cmd < -258.2
        Te_cmd = -258.2;
        e_int = e_int - e_w * Ts_dt;
    end
    
    % 3. Analytical Smooth MTPA Trajectory
    if abs(Te_cmd) < 1e-3 || dL < 1e-7
        id_mtpa = 0.0;
        iq_mtpa = Te_cmd / (1.5 * pp * Psi_val);
    else
        iq_lin = Te_cmd / (1.5 * pp * Psi_val);
        id_mtpa = - (dL / (2.0 * Psi_val)) * (iq_lin^2);
        if id_mtpa < -0.45 * I_max
            id_mtpa = -0.45 * I_max;
        end
        
        denom = Psi_val + (Ld_val - Lq_val) * id_mtpa;
        if abs(denom) < 1e-4
            denom = 1e-4;
        end
        iq_mtpa = Te_cmd / (1.5 * pp * denom);
    end
    
    % 4. Analytical Closed-Form Voltage Ellipse Field Weakening
    V_max = (double(Vdc) / sqrt(3.0)) * 0.95;
    omega_e = max(abs(double(omega_m)), 1.0);
    
    Vd_est = -omega_e * Lq_val * iq_mtpa;
    Vq_est = omega_e * Ld_val * id_mtpa + omega_e * Psi_val;
    V_est = sqrt(Vd_est^2 + Vq_est^2);
    
    if V_est > V_max && omega_e > 2000.0
        V_lim = V_max / omega_e;
        max_iq_sq = max(0.0, (V_lim^2) / (Lq_val^2));
        if (iq_mtpa^2) > 0.90 * max_iq_sq
            iq_fw = sign(iq_mtpa) * sqrt(0.90 * max_iq_sq);
        else
            iq_fw = iq_mtpa;
        end
        
        val_under_sqrt = max(0.0, V_lim^2 - (Lq_val * iq_fw)^2);
        id_fw = (-Psi_val + sqrt(val_under_sqrt)) / Ld_val;
        if id_fw > id_mtpa
            id_fw = (-Psi_val - sqrt(val_under_sqrt)) / Ld_val;
        end
        id_out = id_fw;
        iq_out = iq_fw;
    else
        id_out = id_mtpa;
        iq_out = iq_mtpa;
    end
    
    % 5. Stator Current Circle Clamp
    I_tot = sqrt(id_out^2 + iq_out^2);
    if I_tot > I_max
        id_out = id_out * (I_max / I_tot);
        iq_out = iq_out * (I_max / I_tot);
    end
    
    id_ref(1) = id_out;
    iq_ref(1) = iq_out;
end

== matlab function PMSM_CascadedMPC/AutoTuner ==
  settings: updateMethod=DISCRETE  sampleTime=Ts_ctrl
  data: Rs_est output size=1; Ld_est output size=1; Lq_est output size=1; PsiPM_est output size=1; id_in input; iq_in input; omega_e_in input; vq_ref_in input; omega_ref_ext_in input; Vdc_in input; ctrl_mode output; da output; db output; dc output; omega_ref_out output; J_est output; B_est output; theta_e_in input
function [Rs_est, Ld_est, Lq_est, PsiPM_est, ctrl_mode, da, db, dc, omega_ref_out, J_est, B_est] = ...
    AutoTuner(id_in, iq_in, omega_e_in, vq_ref_in, omega_ref_ext_in, Vdc_in, theta_e_in)
    
    % ====================================================================
    % 1. USER CONFIGURATION BLOCK
    % ====================================================================
    I_MAX_RATING = 565.0;  % Peak phase current of the motor (Amps)
    V_DC_NOMINAL = 400.0;  % Nominal DC link voltage (Volts)
    W_MIN_FLUX   = 800.0;  % Speed required for clean Back-EMF reading
    POLE_PAIRS   = 6.0;    % REQUIRED FOR MECHANICAL MATH: Number of pole pairs
    
    I_SPIN_FLUX = 0.10 * I_MAX_RATING; 
    V_HF_AMP    = 0.04 * V_DC_NOMINAL; 
    % ====================================================================
    persistent state sub_state count state_timer
    persistent int_err_d int_err_q
    persistent Rs_val Ld_val Lq_val PsiPM_val J_val B_val
    persistent V_sum I_sum sample_k 
    persistent Vd1 Id1 I_sin I_cos
    persistent Kp_calc Ki_calc 
    persistent Vd_bias 
    
    % Mechanical estimation persistent variables
    persistent w_start w_start_sum int_err_spd Te_1 w_1
    
    % --- Explicitly initialize outputs for Simulink Coder ---
    Rs_est = 0.0; Ld_est = 0.0; Lq_est = 0.0; PsiPM_est = 0.0;
    ctrl_mode = 0.0; da = 0.0; db = 0.0; dc = 0.0;
    omega_ref_out = 0.0; J_est = 0.0; B_est = 0.0;
    
    Ts = 1e-4;   % Sample time (10 kHz)
    f_hf = 500;  
    w_hf = 2 * pi * f_hf;
    
    if isempty(state)
        state = 0; sub_state = 0; count = 0; state_timer = 0; 
        int_err_d = 0; int_err_q = 0;
        Rs_val = 0.005; Ld_val = 0.0001; Lq_val = 0.0001; PsiPM_val = 0.04;
        J_val = 0.0; B_val = 0.0; 
        V_sum = 0; I_sum = 0; sample_k = 0; 
        Vd1 = 0; Id1 = 0; I_sin = 0; I_cos = 0;
        Kp_calc = 0.1; Ki_calc = 10; 
        Vd_bias = 0;
        w_start = 0; w_start_sum = 0; int_err_spd = 0; Te_1 = 0; w_1 = 0;
    end
    
    t = double(count) * Ts;
    id = double(id_in); iq = double(iq_in); omega_e = double(omega_e_in); 
    Vdc = double(Vdc_in); theta_e = double(theta_e_in);
    omega_ref_ext = double(omega_ref_ext_in);
    
    Vd_applied = 0; Vq_applied = 0;
    
    V_limit = Vdc / 1.5; 
    if V_limit < 1, V_limit = 24; end 
    %% --- DYNAMIC STATE MACHINE ---
    
    if state == 0 % --- STATE 0: Pulse Test for Dynamic PI Tuning ---
        ctrl_mode = 2; 
        
        V_pulse = V_HF_AMP; 
        Vd_applied = V_pulse;
        Vq_applied = 0;
        
        if sample_k == 0
            Id1 = id; 
        end
        
        sample_k = sample_k + 1;
        
        if sample_k >= 5 
            di = id - Id1;
            dt = 5 * Ts;
            
            if di < 0.1, di = 0.1; end 
            
            L_rough = (V_pulse * dt) / di;
            omega_bw = 1000; 
            
            Kp_calc = L_rough * omega_bw;
            Ki_calc = Kp_calc * 100; 
            
            if Kp_calc > 2.0, Kp_calc = 2.0; end
            if Kp_calc < 0.001, Kp_calc = 0.001; end
            
            state = 1; sub_state = 0; state_timer = t;
            sample_k = 0; V_sum = 0; I_sum = 0; Id1 = 0;
        end
        
    elseif state == 1 % --- Identify Stator Resistance (Rs) ---
        ctrl_mode = 2; 
        iq_ref = 0;
        
        if sub_state == 0
            id_ref = 0.10 * I_MAX_RATING; 
            
            err_d = id_ref - id; err_q = iq_ref - iq;
            int_err_d = max(min(int_err_d + err_d * Ts, V_limit/Ki_calc), -V_limit/Ki_calc);
            int_err_q = max(min(int_err_q + err_q * Ts, V_limit/Ki_calc), -V_limit/Ki_calc);
            
            Vd_applied = Kp_calc * err_d + Ki_calc * int_err_d;
            Vq_applied = Kp_calc * err_q + Ki_calc * int_err_q;
            
            if (t - state_timer) > 0.4
                V_sum = V_sum + Vd_applied;
                I_sum = I_sum + id;
                sample_k = sample_k + 1;
            end
            
            if sample_k >= 100
                Vd1 = V_sum / sample_k;
                Id1 = I_sum / sample_k;
                sub_state = 1; state_timer = t;
                V_sum = 0; I_sum = 0; sample_k = 0;
            end
            
        elseif sub_state == 1
            id_ref = 0.20 * I_MAX_RATING; 
            
            err_d = id_ref - id; err_q = iq_ref - iq;
            int_err_d = max(min(int_err_d + err_d * Ts, V_limit/Ki_calc), -V_limit/Ki_calc);
            int_err_q = max(min(int_err_q + err_q * Ts, V_limit/Ki_calc), -V_limit/Ki_calc);
            
            Vd_applied = Kp_calc * err_d + Ki_calc * int_err_d;
            Vq_applied = Kp_calc * err_q + Ki_calc * int_err_q;
            
            if (t - state_timer) > 0.4
                V_sum = V_sum + Vd_applied;
                I_sum = I_sum + id;
                sample_k = sample_k + 1;
            end
            
            if sample_k >= 100
                Vd2 = V_sum / sample_k;
                Id2 = I_sum / sample_k;
                if abs(Id2 - Id1) > 1.0
                    Rs_val = (Vd2 - Vd1) / (Id2 - Id1); if Rs_val < 0.0001, Rs_val = 0.0001; end 
                end
                state = 2; state_timer = t; sub_state = 0;
                int_err_d = 0; int_err_q = 0;
                V_sum = 0; I_sum = 0; sample_k = 0;
            end
        end
        
    elseif state == 2 % --- Identify d-axis Inductance (Ld) ---
        ctrl_mode = 2; 
        
        iq_ref = 0;
        err_q = iq_ref - iq;
        int_err_q = max(min(int_err_q + err_q * Ts, V_limit/Ki_calc), -V_limit/Ki_calc);
        Vq_applied = Kp_calc * err_q + Ki_calc * int_err_q; 
        
        if sub_state == 0
            id_ref = 0.10 * I_MAX_RATING;
            err_d = id_ref - id;
            int_err_d = max(min(int_err_d + err_d * Ts, V_limit/Ki_calc), -V_limit/Ki_calc);
            Vd_applied = Kp_calc * err_d + Ki_calc * int_err_d;
            
            if (t - state_timer) > 0.4
                Vd_bias = Vd_applied; 
                sub_state = 1;
                state_timer = t;
                sample_k = 0; I_sin = 0; I_cos = 0;
            end
            
        elseif sub_state == 1
            Vd_applied = Vd_bias + V_HF_AMP * sin(w_hf * t);
            
            if (t - state_timer) > 0.2
                I_sin = I_sin + id * sin(w_hf * t);
                I_cos = I_cos + id * cos(w_hf * t);
                sample_k = sample_k + 1;
            end
            
            if sample_k >= 200
                I_hf_amp = (2 * sqrt(I_sin^2 + I_cos^2)) / sample_k;
                
                if I_hf_amp > 0.01 
                    Z = V_HF_AMP / I_hf_amp;
                    if Z > Rs_val, Ld_val = sqrt(max(0, Z^2 - Rs_val^2)) / w_hf;
                    else,          Ld_val = Z / w_hf; end
                end
                state = 3; state_timer = t; sub_state = 0;
                int_err_d = 0; int_err_q = 0; 
                I_sin = 0; I_cos = 0; sample_k = 0;
            end
        end
        
    elseif state == 3 % --- Identify q-axis Inductance (Lq) ---
        ctrl_mode = 2; 
        id_ref = 0;
        
        err_d = id_ref - id;
        int_err_d = max(min(int_err_d + err_d * Ts, V_limit/Ki_calc), -V_limit/Ki_calc);
        
        Vd_applied = Kp_calc * err_d + Ki_calc * int_err_d;
        Vq_applied = V_HF_AMP * sin(w_hf * t);
        
        if (t - state_timer) > 0.2
            I_sin = I_sin + iq * sin(w_hf * t);
            I_cos = I_cos + iq * cos(w_hf * t);
            sample_k = sample_k + 1;
        end
        
        if sample_k >= 200
            I_hf_amp = (2 * sqrt(I_sin^2 + I_cos^2)) / sample_k;
            
            if I_hf_amp > 0.01
                Z = V_HF_AMP / I_hf_amp;
                if Z > Rs_val, Lq_val = sqrt(max(0, Z^2 - Rs_val^2)) / w_hf;
                else,          Lq_val = Z / w_hf; end
            end
            state = 4; state_timer = t; sub_state = 0;
            int_err_d = 0; int_err_q = 0; 
            I_sin = 0; I_cos = 0; sample_k = 0; V_sum = 0;
        end
        
    elseif state == 4 % --- Identify PM Flux Linkage (PsiPM) ---
        ctrl_mode = 2; 
        
        if sub_state == 0
            id_ref = 0; 
            iq_ref = I_SPIN_FLUX; 
            
            err_d = id_ref - id; err_q = iq_ref - iq;
            int_err_d = max(min(int_err_d + err_d * Ts, V_limit/Ki_calc), -V_limit/Ki_calc);
            int_err_q = max(min(int_err_q + err_q * Ts, V_limit/Ki_calc), -V_limit/Ki_calc);
            
            Vd_applied = Kp_calc * err_d + Ki_calc * int_err_d;
            Vq_applied = Kp_calc * err_q + Ki_calc * int_err_q;
            
            if abs(omega_e) > W_MIN_FLUX
                sub_state = 1; 
                state_timer = t; 
            end
            
        elseif sub_state == 1
            id_ref = 0; 
            iq_ref = 0; 
            
            err_d = id_ref - id; err_q = iq_ref - iq;
            int_err_d = max(min(int_err_d + err_d * Ts, V_limit/Ki_calc), -V_limit/Ki_calc);
            int_err_q = max(min(int_err_q + err_q * Ts, V_limit/Ki_calc), -V_limit/Ki_calc);
            
            Vd_applied = Kp_calc * err_d + Ki_calc * int_err_d;
            Vq_applied = Kp_calc * err_q + Ki_calc * int_err_q;
            
            if (t - state_timer) > 0.5
                if abs(omega_e) > (W_MIN_FLUX / 2) 
                    inst_psi = Vq_applied / omega_e;
                    V_sum = V_sum + inst_psi;
                    sample_k = sample_k + 1;
                end
            end
            
            if sample_k >= 200
                PsiPM_val = V_sum / sample_k;
                state = 5; sub_state = 0; state_timer = t; 
                sample_k = 0; I_sum = 0; w_start_sum = 0; 
                int_err_spd = 0;
            end
        end
        
    elseif state == 5 % --- Identify Friction (B) and Inertia (J) [Two-Point Method] ---
        ctrl_mode = 2; 
        
        if sub_state == 0 % Point 1: Settle at 60 rad/s
            w_mech = omega_e / POLE_PAIRS;
            w_target = 60.0; 
            
            % Automatically scale PI gains based on the motor's power class
            Kp_spd = 0.005 * I_MAX_RATING; 
            Ki_spd = 0.020 * I_MAX_RATING; 
            
            err_spd = w_target - w_mech;
            int_err_spd = max(min(int_err_spd + err_spd * Ts, I_SPIN_FLUX/Ki_spd), -I_SPIN_FLUX/Ki_spd);
            
            iq_ref = Kp_spd * err_spd + Ki_spd * int_err_spd;
            iq_ref = max(min(iq_ref, I_SPIN_FLUX), -I_SPIN_FLUX); 
            id_ref = 0; 
            
            err_d = id_ref - id; err_q = iq_ref - iq;
            int_err_d = max(min(int_err_d + err_d * Ts, V_limit/Ki_calc), -V_limit/Ki_calc);
            int_err_q = max(min(int_err_q + err_q * Ts, V_limit/Ki_calc), -V_limit/Ki_calc);
            
            Vd_applied = Kp_calc * err_d + Ki_calc * int_err_d;
            Vq_applied = Kp_calc * err_q + Ki_calc * int_err_q;
            
            % STRICT ABSOLUTE TIMER: Wait 1.5s to guarantee acceleration is identically zero.
            if (t - state_timer) > 1.5
                sample_k = sample_k + 1;
                
                % Use the mathematically clean commanded current (iq_ref), not noisy feedback
                I_sum = I_sum + iq_ref; 
                w_start_sum = w_start_sum + w_mech;
                
                if sample_k >= 250 
                    iq_avg = I_sum / 250.0;
                    w_1 = w_start_sum / 250.0;
                    Te_1 = 1.5 * POLE_PAIRS * PsiPM_val * iq_avg;
                    
                    sub_state = 1; state_timer = t; 
                    sample_k = 0; I_sum = 0; w_start_sum = 0; 
                    int_err_spd = 0; int_err_q = 0;
                end
            end
            
        elseif sub_state == 1 % Point 2: Settle at 120 rad/s
            w_mech = omega_e / POLE_PAIRS;
            w_target = 120.0; 
            
            Kp_spd = 0.005 * I_MAX_RATING; 
            Ki_spd = 0.020 * I_MAX_RATING; 
            
            err_spd = w_target - w_mech;
            int_err_spd = max(min(int_err_spd + err_spd * Ts, I_SPIN_FLUX/Ki_spd), -I_SPIN_FLUX/Ki_spd);
            
            iq_ref = Kp_spd * err_spd + Ki_spd * int_err_spd;
            iq_ref = max(min(iq_ref, I_SPIN_FLUX), -I_SPIN_FLUX); 
            id_ref = 0; 
            
            err_d = id_ref - id; err_q = iq_ref - iq;
            int_err_d = max(min(int_err_d + err_d * Ts, V_limit/Ki_calc), -V_limit/Ki_calc);
            int_err_q = max(min(int_err_q + err_q * Ts, V_limit/Ki_calc), -V_limit/Ki_calc);
            
            Vd_applied = Kp_calc * err_d + Ki_calc * int_err_d;
            Vq_applied = Kp_calc * err_q + Ki_calc * int_err_q;
            
            % STRICT ABSOLUTE TIMER: Wait 1.5s to guarantee acceleration is identically zero.
            if (t - state_timer) > 1.5
                sample_k = sample_k + 1;
                
                % Use the mathematically clean commanded current (iq_ref)
                I_sum = I_sum + iq_ref; 
                w_start_sum = w_start_sum + w_mech;
                
                if sample_k >= 250 
                    iq_avg = I_sum / 250.0;
                    w_2 = w_start_sum / 250.0;
                    Te_2 = 1.5 * POLE_PAIRS * PsiPM_val * iq_avg;
                    
                    if abs(w_2 - w_1) > 10.0
                        B_val = abs(Te_2 - Te_1) / abs(w_2 - w_1); 
                    end
                    
                    if B_val <= 0, B_val = 0.0001; end 
                    
                    sub_state = 2; state_timer = t; 
                    sample_k = 0; int_err_q = 0; int_err_spd = 0;
                end
            end
            
        elseif sub_state == 2 % Point 3: Active Braking Step (Identify Inertia J)
            id_ref = 0; 
            iq_ref = -I_SPIN_FLUX; 
            
            err_d = id_ref - id; err_q = iq_ref - iq;
            int_err_d = max(min(int_err_d + err_d * Ts, V_limit/Ki_calc), -V_limit/Ki_calc);
            int_err_q = max(min(int_err_q + err_q * Ts, V_limit/Ki_calc), -V_limit/Ki_calc);
            
            Vd_applied = Kp_calc * err_d + Ki_calc * int_err_d;
            Vq_applied = Kp_calc * err_q + Ki_calc * int_err_q;
            
            if (t - state_timer) > 0.1
                if sample_k == 0
                    w_start = omega_e / POLE_PAIRS;
                end
                
                sample_k = sample_k + 1;
                
                if sample_k >= 100
                    w_end = omega_e / POLE_PAIRS;
                    dw_dt = (w_end - w_start) / (100 * Ts);
                    w_avg = (w_end + w_start) / 2;
                    
                    % Use the clean commanded current for the torque calculation
                    Te = 1.5 * POLE_PAIRS * PsiPM_val * iq_ref;
                    
                    if abs(dw_dt) > 1e-4
                        J_val = abs(Te - (B_val * w_avg)) / abs(dw_dt); 
                    else
                        J_val = 0.0867; 
                    end
                    
                    if J_val <= 0.0001, J_val = 0.001; end 
                    
                    state = 6; 
                end
            end
        end
        
    elseif state == 6 % --- Mission Profile ---
        ctrl_mode = 1; 
        da = 0.5; db = 0.5; dc = 0.5; 
        omega_ref_out = omega_ref_ext;
    end
    
    %% --- INVERSE PARK & SPACE VECTOR MODULATION ---
    if state < 6
        valpha = Vd_applied * cos(theta_e) - Vq_applied * sin(theta_e);
        vbeta  = Vd_applied * sin(theta_e) + Vq_applied * cos(theta_e);
        
        va = valpha; 
        vb = -0.5 * valpha + 0.8660254 * vbeta; 
        vc = -0.5 * valpha - 0.8660254 * vbeta;
        
        voff = -0.5 * (max([va, vb, vc]) + min([va, vb, vc]));
        
        da = (va + voff) / (Vdc / 2) * 0.5 + 0.5;
        db = (vb + voff) / (Vdc / 2) * 0.5 + 0.5;
        dc = (vc + voff) / (Vdc / 2) * 0.5 + 0.5;
        
        da = max(min(da, 1), 0);
        db = max(min(db, 1), 0);
        dc = max(min(dc, 1), 0);
    end
    
    %% --- OUTPUT ASSIGNMENT ---
    Rs_est = Rs_val; 
    Ld_est = Ld_val; 
    Lq_est = Lq_val; 
    PsiPM_est = PsiPM_val;
    J_est = J_val; 
    B_est = B_val;
    
    count = count + 1;
end
